simulink model "Subsystem"  (R2020b)
settings: Solver=VariableStepAuto  StartTime=0.0  StopTime=100  RelTol=1e-3
values from neighbouring files (symbols this model uses):
  b = 50    [parametersCalling.m]
  k1 = 5    [parametersCalling.m]
  k2 = 2    [parametersCalling.m]
  m1 = 100    [parametersCalling.m]
  m2 = 50    [parametersCalling.m]
settings Model: Creator=baner  LastModifiedBy=baner
settings DataIOCC: SaveOutput=off  SaveTime=off

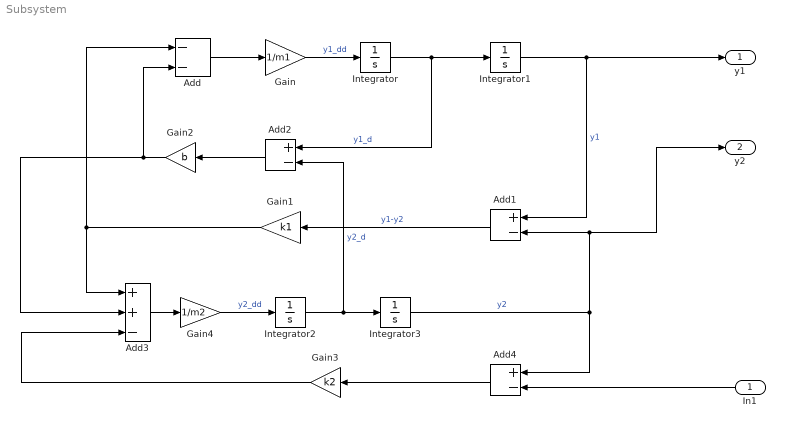
== system Subsystem ==
  In1 : Inport  OutDataTypeStr=double  PortDimensions=1  SampleTime=0
  Add : Sum  Inputs=--
  Add1 : Sum  Inputs=+-
  Add2 : Sum  Inputs=+-
  Add3 : Sum  Inputs=++-
  Add4 : Sum  Inputs=+-
  Gain : Gain  Gain=1/m1
  Gain1 : Gain  Gain=k1
  Gain2 : Gain  Gain=b
  Gain3 : Gain  Gain=k2
  Gain4 : Gain  Gain=1/m2
  Integrator{,1..3} (4 alike) : Integrator
  y1 : Outport  OutDataTypeStr=double  PortDimensions=1  SampleTime=0
  y2 : Outport  Port=2  OutDataTypeStr=double  PortDimensions=1  SampleTime=0
  wires:
  Integrator3/1 -> Add4/1, Add1/2, y2/1  "y2"
  Integrator/1 -> Integrator1/1, Add2/1  "y1_d"
  Add3/1 -> Gain4/1
  Integrator1/1 -> Add1/1, y1/1  "y1"
  Gain1/1 -> Add/1, Add3/1
  Integrator2/1 -> Integrator3/1, Add2/2  "y2_d"
  Add/1 -> Gain/1
  Gain/1 -> Integrator/1  "y1_dd"
  Add1/1 -> Gain1/1  "y1-y2"
  Gain3/1 -> Add3/3
  Gain2/1 -> Add/2, Add3/2
  Gain4/1 -> Integrator2/1  "y2_dd"
  Add2/1 -> Gain2/1
  Add4/1 -> Gain3/1
  In1/1 -> Add4/2
